simulink model "open_loop_bldc_motor"  (R2024a)
settings: Solver=VariableStepAuto  StartTime=0.0  StopTime=10  RelTol=1e-3
undefined symbols (not defined in the file): ts
libraries: simulink x7, spsDCVoltageSourceLib x1, spsPermanentMagnetSynchronousMachineLib x1, spsUniversalBridgeLib x1, spsVoltageMeasurementLib x1, sps_lib x1
settings Model: Creator=HP  LastModifiedBy=HP

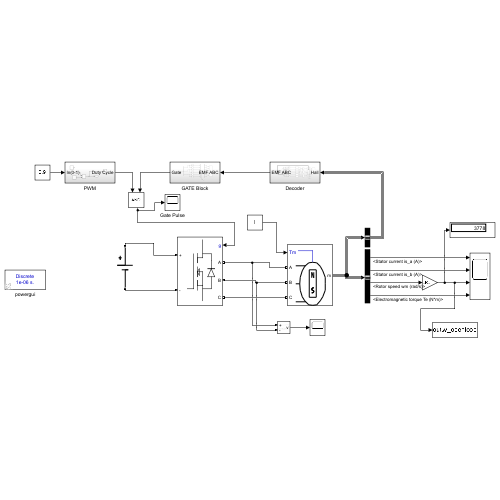
[thumbnail: Simulink's stored preview of the top-level diagram]
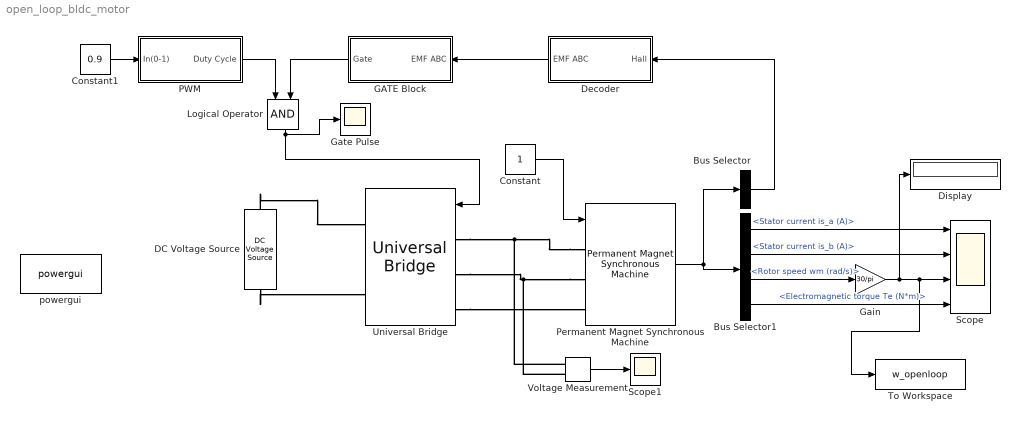
== system open_loop_bldc_motor ==
  Bus Selector : BusSelector  OutputSignals=Hall effect signal h_a,Hall effect signal h_b,Hall effect signal h_c  OutputAsBus=on
  Bus Selector1 : BusSelector  OutputSignals=Stator current is_a (A),Stator current is_b (A),Rotor speed wm (rad/s),Electromagnetic torque Te (N*m)
  Constant : Constant
  Constant1 : Constant  Value=0.9
  DC Voltage Source : spsDCVoltageSourceLib/DC Voltage Source  Amplitude=500  Measurements=None
  Decoder : Subsystem
  Display : Display
  GATE Block : Subsystem
  Gain : Gain  Gain=30/pi
  Gate Pulse : Scope
  Logical Operator : Logic  AllPortsSameDT=off  OutDataTypeStr=boolean
  PWM : Subsystem
  Permanent Magnet Synchronous Machine : spsPermanentMagnetSynchronousMachineLib/Permanent Magnet Synchronous Machine  NbPhases=3  FluxDistribution=Trapezoidal  RotorType=Round  MechanicalLoad=Torque Tm  PresetModel=No  ShowDetailedParameters=on  MeasurementBus=off  Resistance=0.0485  Inductance=8.5e-3  dqInductances=[8.5e-3,8.5e-3]  La=0.000395  MachineConstant=Flux linkage established by magnets (V.s)  Flux=0.1194  VoltageCst=100.0283  TorqueCst=0.9552  Flat=120  Mechanical=[0.0027 0.0004924 4 0]  PolePairs=4  InitialConditions=[0,0, 0,0]  InitialConditions5ph=[0 0 0 0 0 0]  RefAngle=90 degrees behind phase A axis (modified Park)  IterativeDiscreteModel=Trapezoidal non iterative  TsBlock=-1  TsPowergui=0
  Scope : Scope  NumInputPorts=4
  Scope1 : Scope
  To Workspace : ToWorkspace  VariableName=w_openloop  SampleTime=-1
  Universal Bridge : spsUniversalBridgeLib/Universal Bridge  Arms=3  SnubberResistance=1e5  SnubberCapacitance=inf  Device=MOSFET / Diodes  Ron=1e-3  Lon=0  ForwardVoltages="[  0  0  ]"  ForwardVoltage=0  GTOparameters=[ 10e-6 , 20e-6 ]  IGBTparameters=[ 1e-6 , 2e-6 ]  Measurements=None  Measurements_2=None  converterType=Rectifier
  Voltage Measurement : spsVoltageMeasurementLib/Voltage Measurement  PhasorSimulation=off  OutputType=Complex  PSBequivalent=0
  powergui : sps_lib/powergui  Priority=1  SimulationMode=Discrete  SampleTime=ts  frequency=60  Iterations=50  frequencyindice=0  Pbase=100e6  ErrMax=1e-4  UnitsV=kV  UnitsW=MW  buscounter=0  FunctionMessages=off  echomessages=off  EnableUseOfTLC=off  CurrentSourceSwitches=off  DisableSnubberDevices=off  DisableRonSwitches=off  DisableVfSwitches=off  DisplayEquations=off  AutomaticDiscreteSolvers=off  SolverType=Tustin/Backward Euler (TBE)  Interpol=off  ExternalGateDelay=off  methode=off  Ts=100  x0status=blocks  SPID=on  SwTol=0  HookPort=off  NonlinearTolerance=1e-4  nMaxIteration=100  ContinueOnMaxIteration=off  RestoreLinks=warning  ResistiveCurrentMeasurement=off  Frange=[0:2:500]  Ylog=off  Xlog=on  ShowGrid=off  save=off  variable=ZData  structure=0  ZoomFFT=off  StartTime=0.0  cycles=1  DisplayStyle=1  fundamental=60  FreqAxis=off  MaxFrequency=1000  frequencyindicesteady=1  RmsSteady=1  display=off
  wires:
  Gain/1 -> Display/1, To Workspace/1, Scope/3
  Bus Selector1/3 -> Gain/1  "<Rotor speed wm (rad/s)>"
  Bus Selector/1 -> Decoder/1(Hall)
  Voltage Measurement/1 -> Scope1/1
  PWM/1(Duty Cycle) -> Logical Operator/1
  Logical Operator/1 -> Universal Bridge/1, Gate Pulse/1
  Decoder/1(EMF ABC) -> GATE Block/1(EMF ABC)
  GATE Block/1(Gate) -> Logical Operator/2
  Permanent Magnet Synchronous Machine/1 -> Bus Selector1/1, Bus Selector/1
  Bus Selector1/4 -> Scope/4  "<Electromagnetic torque Te (N*m)>"
  Bus Selector1/2 -> Scope/2  "<Stator current is_b (A)>"
  Constant/1 -> Permanent Magnet Synchronous Machine/1
  Bus Selector1/1 -> Scope/1  "<Stator current is_a (A)>"
  Constant1/1 -> PWM/1(In(0-1))
  connections:
  Permanent Magnet Synchronous Machine/LConn2 -- Universal Bridge/LConn2 -- Voltage Measurement/LConn2
  Permanent Magnet Synchronous Machine/LConn1 -- Universal Bridge/LConn1 -- Voltage Measurement/LConn1
  Universal Bridge/LConn3 -- Permanent Magnet Synchronous Machine/LConn3
  DC Voltage Source/RConn1 -- Universal Bridge/RConn1
  DC Voltage Source/LConn1 -- Universal Bridge/RConn2

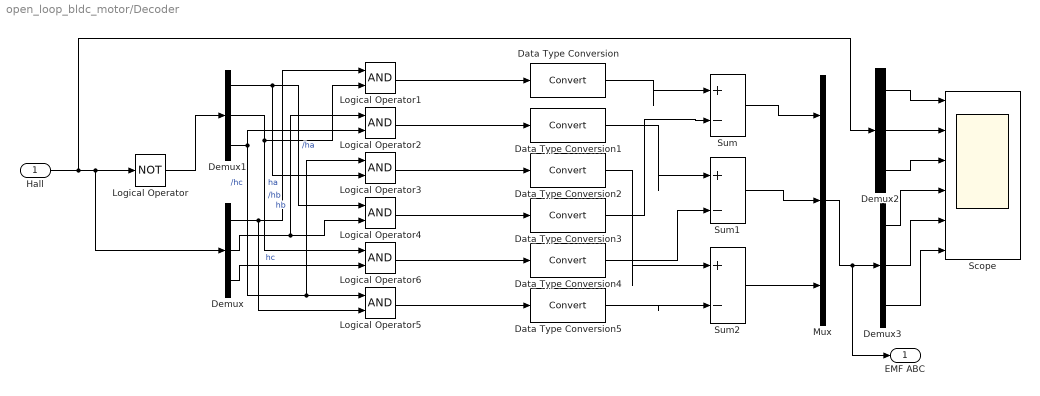
== system open_loop_bldc_motor/Decoder ==
  Hall : Inport
  Data Type Conversion{,1..5} (6 alike) : DataTypeConversion  SaturateOnIntegerOverflow=off  RndMeth=Floor
  Demux{,1..3} (4 alike) : Demux  Outputs=3
  Logical Operator : Logic  Operator=NOT  AllPortsSameDT=off  OutDataTypeStr=boolean
  Logical Operator{1..6} (6 alike) : Logic  AllPortsSameDT=off  OutDataTypeStr=boolean
  Mux : Mux  Inputs=3
  Scope : Scope  NumInputPorts=6
  Sum : Sum  Inputs=|+-
  Sum1 : Sum  Inputs=|+-
  Sum2 : Sum  Inputs=|+-
  EMF ABC : Outport
  wires:
  Hall/1 -> Demux2/1, Demux/1, Logical Operator/1
  Logical Operator/1 -> Demux1/1
  Logical Operator1/1 -> Data Type Conversion/1
  Logical Operator2/1 -> Data Type Conversion1/1
  Logical Operator3/1 -> Data Type Conversion2/1
  Logical Operator4/1 -> Data Type Conversion3/1
  Logical Operator6/1 -> Data Type Conversion4/1
  Logical Operator5/1 -> Data Type Conversion5/1
  Data Type Conversion/1 -> Sum/1
  Data Type Conversion1/1 -> Sum1/1
  Data Type Conversion2/1 -> Sum2/1
  Data Type Conversion3/1 -> Sum/2
  Data Type Conversion4/1 -> Sum1/2
  Data Type Conversion5/1 -> Sum2/2
  Sum/1 -> Mux/1
  Sum1/1 -> Mux/2
  Sum2/1 -> Mux/3
  Mux/1 -> EMF ABC/1, Demux3/1
  Demux2/1 -> Scope/1
  Demux2/2 -> Scope/2
  Demux2/3 -> Scope/3
  Demux3/1 -> Scope/4
  Demux3/2 -> Scope/5
  Demux3/3 -> Scope/6
  Demux1/1 -> Logical Operator3/2, Logical Operator4/1  "/ha"
  Demux1/2 -> Logical Operator1/2, Logical Operator6/1  "/hb"
  Demux1/3 -> Logical Operator3/1, Logical Operator5/1, Logical Operator2/2  "/hc"
  Demux/1 -> Logical Operator5/2, Logical Operator1/1  "ha"
  Demux/2 -> Logical Operator2/1, Logical Operator4/2  "hb"
  Demux/3 -> Logical Operator6/2  "hc"

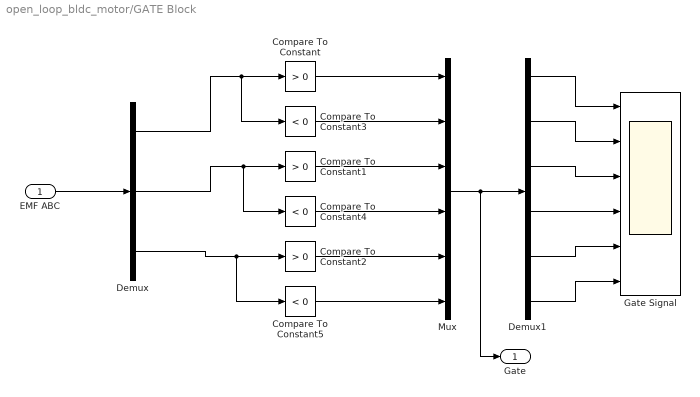
== system open_loop_bldc_motor/GATE Block ==
  EMF ABC : Inport
  Compare To Constant : simulink/Logic and Bit Operations/Compare To Constant  relop=>  const=0  OutDataTypeStr=boolean
  Compare To Constant1 : simulink/Logic and Bit Operations/Compare To Constant  relop=>  const=0  OutDataTypeStr=boolean
  Compare To Constant2 : simulink/Logic and Bit Operations/Compare To Constant  relop=>  const=0  OutDataTypeStr=boolean
  Compare To Constant3 : simulink/Logic and Bit Operations/Compare To Constant  relop=<  const=0  OutDataTypeStr=boolean
  Compare To Constant4 : simulink/Logic and Bit Operations/Compare To Constant  relop=<  const=0  OutDataTypeStr=boolean
  Compare To Constant5 : simulink/Logic and Bit Operations/Compare To Constant  relop=<  const=0  OutDataTypeStr=boolean
  Demux : Demux  Outputs=3
  Demux1 : Demux  Outputs=6
  Gate Signal : Scope  NumInputPorts=6
  Mux : Mux  Inputs=6
  Gate : Outport
  wires:
  EMF ABC/1 -> Demux/1
  Demux/1 -> Compare To Constant3/1, Compare To Constant/1
  Demux/2 -> Compare To Constant4/1, Compare To Constant1/1
  Demux/3 -> Compare To Constant5/1, Compare To Constant2/1
  Compare To Constant/1 -> Mux/1
  Compare To Constant3/1 -> Mux/2
  Compare To Constant1/1 -> Mux/3
  Compare To Constant4/1 -> Mux/4
  Compare To Constant2/1 -> Mux/5
  Compare To Constant5/1 -> Mux/6
  Mux/1 -> Gate/1, Demux1/1
  Demux1/1 -> Gate Signal/1
  Demux1/2 -> Gate Signal/2
  Demux1/3 -> Gate Signal/3
  Demux1/4 -> Gate Signal/4
  Demux1/5 -> Gate Signal/5
  Demux1/6 -> Gate Signal/6

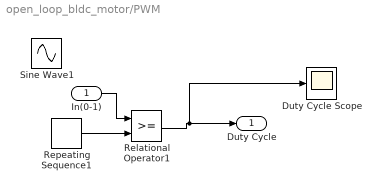
== system open_loop_bldc_motor/PWM ==
  In(0-1) : Inport
  Duty Cycle Scope : Scope
  Relational Operator1 : RelationalOperator  OutDataTypeStr=boolean  RndMeth=Simplest  InputSameDT=off
  Repeating Sequence1 : simulink/Sources/Repeating Sequence  rep_seq_t=[0 50e-6 100e-6]  rep_seq_y=[0 1 0]
  Sine Wave1 : Sin  SampleTime=0
  Duty Cycle : Outport
  wires:
  In(0-1)/1 -> Relational Operator1/1
  Relational Operator1/1 -> Duty Cycle Scope/1, Duty Cycle/1
  Repeating Sequence1/1 -> Relational Operator1/2
